simulink model "State_Machine"  (R2022b)
settings: configuration reference "BMS_Sw_CodeGenConfig" (kept outside this file)
settings Model: DataDictionary=DD_State_Machine.sldd  EnableAccessToBaseWorkspace=off  ExtModeTrigDuration=5  Creator=Chirag Patel  LastModifiedBy=cpatel
settings ConfigSetRef: SourceName=BMS_Sw_CodeGenConfig

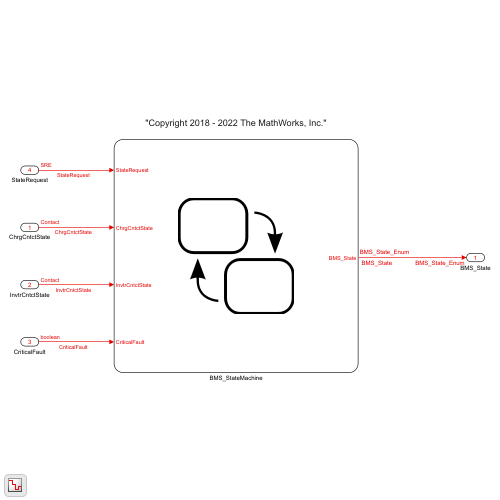
[thumbnail: Simulink's stored preview of the top-level diagram]
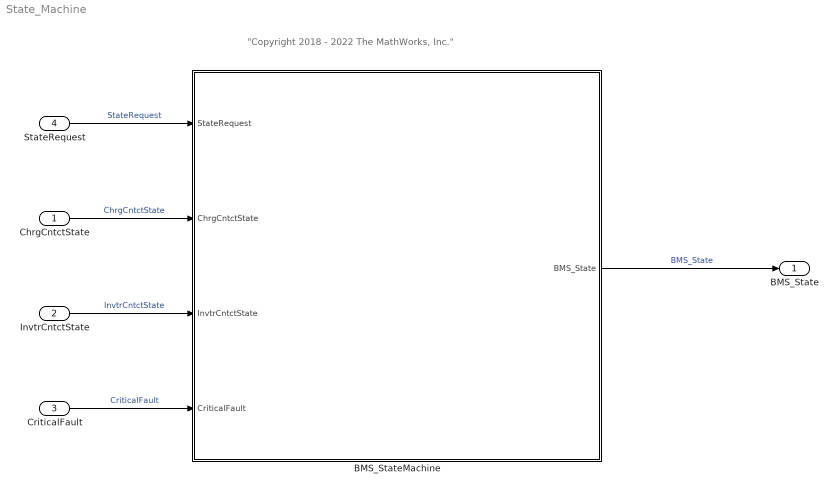
== system State_Machine ==
  note: "Copyright 2018 - 2022 The MathWorks, Inc."
  ChrgCntctState : Inport
  InvtrCntctState : Inport  Port=2
  CriticalFault : Inport  Port=3
  StateRequest : Inport  Port=4  OutDataTypeStr=Enum: SRE  PortDimensions=1  SampleTime=[0.10000000000000001,0]  Interpolate=off
  BMS_StateMachine : Stateflow chart  TreatAsAtomicUnit=on  VariantControl=(default)
  BMS_State : Outport  OutDataTypeStr=Enum: BMS_State_Enum  PortDimensions=1  SampleTime=[0.10000000000000001,0]  VectorParamsAs1DForOutWhenUnconnected=off
  wires:
  BMS_StateMachine/1(BMS_State) -> BMS_State/1  "BMS_State"
  StateRequest/1 -> BMS_StateMachine/1(StateRequest)  "StateRequest"
  ChrgCntctState/1 -> BMS_StateMachine/2(ChrgCntctState)  "ChrgCntctState"
  InvtrCntctState/1 -> BMS_StateMachine/3(InvtrCntctState)  "InvtrCntctState"
  CriticalFault/1 -> BMS_StateMachine/4(CriticalFault)  "CriticalFault"

== stateflow chart State_Machine/BMS_StateMachine ==
  state Driving
    en:
    BMS_State = ...
    BMS_State_Enum.BMS_Driving;
  state Standby
    en:
    BMS_State = ...
    BMS_State_Enum.BMS_Standby;
  state Charging
    en:
    BMS_State = ...
    BMS_State_Enum.BMS_Charging;
  state Fault
    en,du:
    BMS_State = BMS_State_Enum.BMS_Fault;
  (default) -> Standby
  Standby -> Charging [order 1] : [StateRequest ==SRE.Charging...
      | && ChrgCntctState == Contact.Close]
  Standby -> Driving [order 3] : [StateRequest == SRE.Driving && ...
      | InvtrCntctState == Contact.Close]
  Charging -> Standby [order 2] : [StateRequest ~=SRE.Charging...
      | || ChrgCntctState ~= Contact.Close]
  Driving -> Standby [order 2] : [StateRequest ~= SRE.Driving || ...
      | InvtrCntctState ~= Contact.Close]
  Driving -> Fault [order 1] : [CriticalFault]
  Standby -> Fault [order 2] : [CriticalFault]
  Fault -> Standby : [~CriticalFault]
  Charging -> Fault [order 1] : [CriticalFault]
  data: StateRequest input Enum: SRE; BMS_State output Enum: BMS_State_Enum =BMS_State_Enum.BMS_Standby; ChrgCntctState input Enum: Contact; InvtrCntctState input Enum: Contact; CriticalFault input boolean
